simulink model "Opera_Delt_Angulos"  (R2014a)
settings: Solver=ode45  StartTime=0.0  StopTime=1  RelTol=1e-3
PreLoadFcn:
  | Fs=0.001;
  | Fc=0.0005;
InitFcn:
  | Fs=0.001;
  | Fc=0.0005;
undefined symbols (not defined in the file or in its folder): X, Y, Z
libraries: sm_lib x238, Fricciones x12, nesl_utility x10, powerlib x1
(part 1 of 5)
Description:
  | Modelo de un robot tipo Delta, con:
  | -Fricción en las articulaciones
  | -Con interpolador de orden 5 en el espacio operacional.
  | -Cinematica inversa
  | -Sigue una trayectoria dada de pick and place, y devuelve los torques.
settings Model: Creator=Sebastian Serna Palleja  LastModifiedBy=Sebastian
settings Model: ModifiedComment=|
  | Sebastian -- Mon Apr 11 18:42:01 2016 -- Version 1.108
  | Actualizacion pesos
settings Model: ModifiedHistory=|
  | Sebastian -- Mon Apr 11 18:42:01 2016 -- Version 1.108
  | Actualizacion pesos
  | 
  | Modelo con funcion de pick and place,
  | organizado, con interpolador en el espacio operacional de orden 5.
settings SolverCC: ConsecutiveZCsStepRelTol=10*100*eps  ZeroCrossControl=EnableAll  AutoInsertRateTranBlk=on

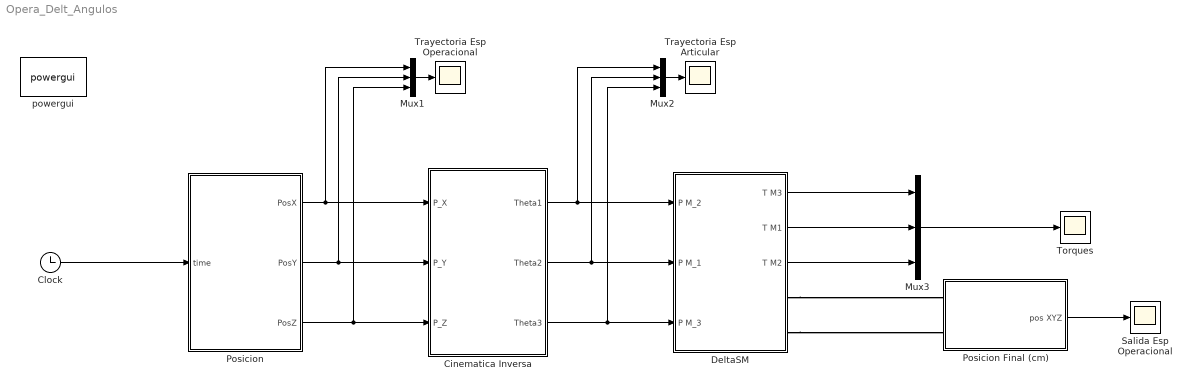
== system Opera_Delt_Angulos ==
  Cinematica Inversa : Subsystem
  Clock : Clock
  DeltaSM : Subsystem
  Mux1 : Mux  Inputs=3
  Mux2 : Mux  Inputs=3
  Mux3 : Mux  Inputs=3
  "Posicion " : MATLAB Function  TreatAsAtomicUnit=on
  Posicion Final (cm) : Subsystem
  Salida Esp Operacional : Scope
      settings: SaveName=ScopeData5
  Torques : Scope
      settings: YMin=-0.25  YMax=0.225  SaveName=Torque
  Trayectoria Esp Articular : Scope
      settings: SaveName=ScopeData4
  Trayectoria Esp Operacional : Scope
      settings: SaveName=ScopeData3
  powergui : powerlib/powergui  Priority=1  SimulationMode=Continuous  SolverType=Tustin  SampleTime=50e-6  frequency=60  SPID=off  DisableSnubberDevices=off  DisableRonSwitches=off  DisableVfSwitches=off  SwTol=0  Interpol=off  DisplayEquations=off  Ts=0  methode=off  frequencyindice=60  Pbase=100e6  ErrMax=1e-4  Iterations=50  UnitsV=kV  UnitsW=MW  FunctionMessages=off  echomessages=off  HookPort=off  EnableUseOfTLC=off  x0status=blocks  RestoreLinks=warning  ResistiveCurrentMeasurement=off  Frange=[0:2:500]  Ylog=off  Xlog=on  ShowGrid=off  save=off  variable=ZData  structure=0  ZoomFFT=off  StartTime=0.0  cycles=1  DisplayStyle=1  fundamental=60  FreqAxis=off  MaxFrequency=1000  frequencyindicesteady=1  RmsSteady=1  display=off
  wires:
  Posicion Final (cm)/1(pos XYZ) -> Salida Esp Operacional/1
  Clock/1 -> "Posicion "/1(time)
  Mux1/1 -> Trayectoria Esp Operacional/1
  Mux3/1 -> Torques/1
  DeltaSM/2(T M1) -> Mux3/2
  "Posicion "/3(PosZ) -> Mux1/3, Cinematica Inversa/3(P_Z)
  "Posicion "/2(PosY) -> Mux1/2, Cinematica Inversa/2(P_Y)
  "Posicion "/1(PosX) -> Cinematica Inversa/1(P_X), Mux1/1
  Mux2/1 -> Trayectoria Esp Articular/1
  Cinematica Inversa/3(Theta3) -> Mux2/3, DeltaSM/3(P M_3)
  Cinematica Inversa/2(Theta2) -> Mux2/2, DeltaSM/2(P M_1)
  Cinematica Inversa/1(Theta1) -> Mux2/1, DeltaSM/1(P M_2)
  DeltaSM/3(T M2) -> Mux3/3
  DeltaSM/1(T M3) -> Mux3/1
  connections:
  DeltaSM/RConn2 -- Posicion Final (cm)/LConn2
  DeltaSM/RConn1 -- Posicion Final (cm)/LConn1

== system Opera_Delt_Angulos/Cinematica Inversa ==
  P_X : Inport
  P_Y : Inport  Port=2
  P_Z : Inport  Port=3
  Cinematica Inversa : MATLAB Function  TreatAsAtomicUnit=on
  G_1 : Gain
  G_2 : Gain
  G_3 : Gain  Gain=-1
  Retardo1 : TransportDelay  DelayTime=0.01
  Retardo2 : TransportDelay  DelayTime=0.01
  Retardo3 : TransportDelay  DelayTime=0.01
  Theta1 : Outport
  Theta2 : Outport  Port=2
  Theta3 : Outport  Port=3
  wires:
  P_X/1 -> Cinematica Inversa/1(Px)
  P_Y/1 -> Cinematica Inversa/2(Py)
  Cinematica Inversa/3(ThetaM3) -> G_3/1, Retardo1/1
  Cinematica Inversa/1(ThetaM1) -> G_1/1, Retardo3/1
  Retardo2/1 -> Cinematica Inversa/5(AntThetaM2)
  Retardo3/1 -> Cinematica Inversa/4(AntThetaM1)
  Retardo1/1 -> Cinematica Inversa/6(AntThetaM3)
  Cinematica Inversa/2(ThetaM2) -> G_2/1, Retardo2/1
  G_1/1 -> Theta1/1
  G_2/1 -> Theta2/1
  G_3/1 -> Theta3/1
  P_Z/1 -> Cinematica Inversa/3(Pz)

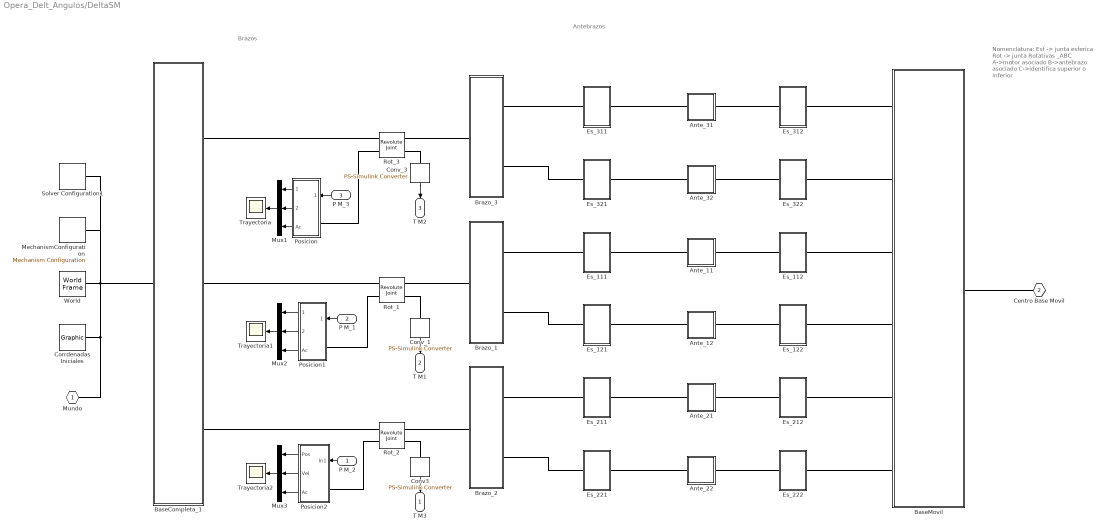
== system Opera_Delt_Angulos/DeltaSM ==
  note: Nomenclatura:
      | Esf  -> junta esferica
      | Rot -> junta Rotativas
      |
      | _ABC
      | A->motor asociado
      | B->antebrazo asociado
      | C->identifica superior o inferior
  note: Brazos
  note: Antebrazos
  P M_2 : Inport
  P M_1 : Inport  Port=2
  P M_3 : Inport  Port=3
  Ante_11 : Subsystem
  Ante_12 : Subsystem
  Ante_21 : Subsystem
  Ante_22 : Subsystem
  Ante_31 : Subsystem
  Ante_32 : Subsystem
  BaseCompleta_1 : Subsystem
  BaseMovil : Subsystem
  Brazo_1 : Subsystem
  Brazo_2 : Subsystem
  Brazo_3 : Subsystem
  Conv3 : nesl_utility/PS-Simulink Converter  PhysicalDomain=network_engine_domain  SubClassName=ps_output  LeftPortType=input  RightPortType=output  PseudoPeriodic=off  Frequencies=[]  Unit=N*m  AffineConversion=off
  Conv_1 : nesl_utility/PS-Simulink Converter  PhysicalDomain=network_engine_domain  SubClassName=ps_output  LeftPortType=input  RightPortType=output  PseudoPeriodic=off  Frequencies=[]  Unit=N*m  AffineConversion=off
  Conv_3 : nesl_utility/PS-Simulink Converter  PhysicalDomain=network_engine_domain  SubClassName=ps_output  LeftPortType=input  RightPortType=output  PseudoPeriodic=off  Frequencies=[]  Unit=N*m  AffineConversion=off
  "Corrdenadas Iniciales " : sm_lib/Body Elements/Graphic  GraphicType=Marker  MarkerShape=Frame  MarkerSize=25  MarkerSizeUnits=m  GraphicVisPropType=SimpleVisualProperties  GraphicDiffuseColor=[0.0 0.0 0.0]  GraphicSpecularColor=[0.2 0.2 0.2]  GraphicAmbientColor=[0.5 0.5 0.5]  GraphicEmissiveColor=[0.0 0.0 0.0 1.0]  GraphicShininess=24.0  GraphicOpacity=1.0  BlockFunction=simmechanics.library.body_elements.graphic
  Es_111 : Subsystem
  Es_112 : Subsystem
  Es_121 : Subsystem
  Es_122 : Subsystem
  Es_211 : Subsystem
  Es_212 : Subsystem
  Es_221 : Subsystem
  Es_222 : Subsystem
  Es_311 : Subsystem
  Es_312 : Subsystem
  Es_321 : Subsystem
  Es_322 : Subsystem
  MechanismConfiguration : sm_lib/Utilities/Mechanism Configuration  UniformGravity=Constant  GravityVector=[0 0 -9.81]  GravityUnits=m/s^2  LinearizationDelta=0.001  BlockFunction=simmechanics.library.utilities.mechanism_configuration
  Mux1 : Mux  Inputs=3
  Mux2 : Mux  Inputs=3
  Mux3 : Mux  Inputs=3
  Posicion : Subsystem
  Posicion1 : Subsystem
  Posicion2 : Subsystem
  Rot_1 : sm_lib/Joints/Revolute Joint  SenseConstraintForce=off  SenseConstraintForceX=off  SenseConstraintForceY=off  SenseConstraintForceZ=off  SenseConstraintTorque=off  SenseConstraintTorqueX=off  SenseConstraintTorqueY=off  SenseConstraintTorqueZ=off  SenseTotalForce=off  SenseTotalForceX=off  SenseTotalForceY=off  SenseTotalForceZ=off  SenseTotalTorque=off  SenseTotalTorqueX=off  SenseTotalTorqueY=off  SenseTotalTorqueZ=off  CompositeWrenchDir=FollowerOnBase  CompositeWrenchFrame=BaseFrame  EquilibriumPosition=0  EquilibriumPositionUnits=rad  SpringStiffness=0  SpringStiffnessUnits=m*N/rad  DampingCoefficient=0  DampingCoefficientUnits=m*s*N/rad  TorqueActuationMode=ComputedTorque  MotionActuationMode=InputMotion  SensePosition=off  SenseVelocity=off  SenseAcceleration=off  SenseTorqueForce=on  PositionTargetValue=-154.29618803259041  PositionTargetValueUnits=deg  PositionTargetSpecify=off  PositionTargetPriority=Low  VelocityTargetValue=0  VelocityTargetValueUnits=deg/s  VelocityTargetSpecify=off  VelocityTargetPriority=High  BlockFunction=simmechanics.library.joints.revolute_joint
  Rot_2 : sm_lib/Joints/Revolute Joint  SenseConstraintForce=off  SenseConstraintForceX=off  SenseConstraintForceY=off  SenseConstraintForceZ=off  SenseConstraintTorque=off  SenseConstraintTorqueX=off  SenseConstraintTorqueY=off  SenseConstraintTorqueZ=off  SenseTotalForce=off  SenseTotalForceX=off  SenseTotalForceY=off  SenseTotalForceZ=off  SenseTotalTorque=off  SenseTotalTorqueX=off  SenseTotalTorqueY=off  SenseTotalTorqueZ=off  CompositeWrenchDir=FollowerOnBase  CompositeWrenchFrame=BaseFrame  EquilibriumPosition=0  EquilibriumPositionUnits=rad  SpringStiffness=0  SpringStiffnessUnits=m*N/rad  DampingCoefficient=0  DampingCoefficientUnits=m*s*N/rad  TorqueActuationMode=ComputedTorque  MotionActuationMode=InputMotion  SensePosition=off  SenseVelocity=off  SenseAcceleration=off  SenseTorqueForce=on  PositionTargetValue=-72.758960975562829  PositionTargetValueUnits=deg  PositionTargetSpecify=off  PositionTargetPriority=Low  VelocityTargetValue=0  VelocityTargetValueUnits=deg/s  VelocityTargetSpecify=off  VelocityTargetPriority=High  BlockFunction=simmechanics.library.joints.revolute_joint
  Rot_3 : sm_lib/Joints/Revolute Joint  SenseConstraintForce=off  SenseConstraintForceX=off  SenseConstraintForceY=off  SenseConstraintForceZ=off  SenseConstraintTorque=off  SenseConstraintTorqueX=off  SenseConstraintTorqueY=off  SenseConstraintTorqueZ=off  SenseTotalForce=off  SenseTotalForceX=off  SenseTotalForceY=off  SenseTotalForceZ=off  SenseTotalTorque=off  SenseTotalTorqueX=off  SenseTotalTorqueY=off  SenseTotalTorqueZ=off  CompositeWrenchDir=FollowerOnBase  CompositeWrenchFrame=BaseFrame  EquilibriumPosition=0  EquilibriumPositionUnits=rad  SpringStiffness=0  SpringStiffnessUnits=m*N/rad  DampingCoefficient=0  DampingCoefficientUnits=m*s*N/rad  TorqueActuationMode=ComputedTorque  MotionActuationMode=InputMotion  SensePosition=off  SenseVelocity=off  SenseAcceleration=off  SenseTorqueForce=on  PositionTargetValue=0  PositionTargetValueUnits=deg  PositionTargetSpecify=off  PositionTargetPriority=Low  VelocityTargetValue=0  VelocityTargetValueUnits=deg/s  VelocityTargetSpecify=off  VelocityTargetPriority=High  BlockFunction=simmechanics.library.joints.revolute_joint
  Solver Configuration1 : nesl_utility/Solver Configuration  PhysicalDomain=network_engine_domain  SubClassName=solver  LeftPortType=input  RightPortType=generic  Accelerate=off  Tones=[]  Harmonics=[]  SimulateNoise=off  Profile=off  UseLocalSampling=off  EnableSwitchedLinearOptims=on  FrequencyDomain=off  UseCCode=off  RelTol=0.001  AbsTol=1e-06  MinStep=1e-09  ToWorkspace=off  DoDC=on  ResidualTolerance=1e-09  UseLocalSolver=on  LocalSolverChoice=NE_BACKWARD_EULER_ADVANCER  LocalSolverSampleTime=0.00005  DoFixedCost=on  MaxNonlinIter=50  MaxModeIter=2  LinearAlgebra=Full  DelaysMemoryBudget=2048  AutomaticFiltering=on  FilteringTimeConstant=0.001
  Trayectoria : Scope
  Trayectoria1 : Scope
      settings: YMin=-3  YMax=0
  Trayectoria2 : Scope
      settings: SaveName=ScopeData2
  World : sm_lib/Frames and Transforms/World Frame  BlockFunction=simmechanics.library.frames_transforms.world_frame
  Mundo : PMIOPort  Port=1  Side=Right
  Centro Base Movil : PMIOPort  Port=2  Side=Right
  T M3 : Outport
  T M1 : Outport  Port=2
  T M2 : Outport  Port=3
  wires:
  Conv_3/1 -> T M2/1
  P M_3/1 -> Posicion/1(In1)
  Mux1/1 -> Trayectoria/1
  Posicion/1(Pos) -> Mux1/1
  Posicion/2(Vel) -> Mux1/2
  Posicion/3(Ac) -> Mux1/3
  Conv_1/1 -> T M1/1
  P M_1/1 -> Posicion1/1(In1)
  Mux2/1 -> Trayectoria1/1
  Posicion1/3(Ac) -> Mux2/3
  Conv3/1 -> T M3/1
  P M_2/1 -> Posicion2/1(In1)
  Mux3/1 -> Trayectoria2/1
  Posicion2/1(Pos) -> Mux3/1
  Posicion2/2(Vel) -> Mux3/2
  Posicion2/3(Ac) -> Mux3/3
  Posicion1/2(Vel) -> Mux2/2
  Posicion1/1(Pos) -> Mux2/1
  connections:
  BaseCompleta_1/RConn2 -- Rot_1/LConn1
  Brazo_2/LConn1 -- Rot_2/RConn1
  BaseCompleta_1/RConn1 -- Rot_3/LConn1
  Brazo_3/LConn1 -- Rot_3/RConn1
  Brazo_1/LConn1 -- Rot_1/RConn1
  BaseCompleta_1/RConn3 -- Rot_2/LConn1
  "Corrdenadas Iniciales "/RConn1 -- Mundo/RConn1 -- BaseCompleta_1/LConn1 -- Solver Configuration1/RConn1 -- MechanismConfiguration/RConn1 -- World/RConn1
  Posicion/LConn1 -- Rot_3/LConn2
  Conv_3/LConn1 -- Rot_3/RConn2
  Posicion1/LConn1 -- Rot_1/LConn2
  Conv_1/LConn1 -- Rot_1/RConn2
  Posicion2/LConn1 -- Rot_2/LConn2
  Conv3/LConn1 -- Rot_2/RConn2
  BaseMovil/RConn1 -- Centro Base Movil/RConn1
  Ante_31/LConn1 -- Es_311/RConn1
  Ante_21/RConn1 -- Es_212/LConn1
  BaseMovil/LConn3 -- Es_112/RConn1
  BaseMovil/LConn2 -- Es_322/RConn1
  Brazo_1/RConn2 -- Es_121/LConn1
  Brazo_3/RConn2 -- Es_321/LConn1
  Ante_21/LConn1 -- Es_211/RConn1
  BaseMovil/LConn6 -- Es_222/RConn1
  Ante_22/LConn1 -- Es_221/RConn1
  Brazo_1/RConn1 -- Es_111/LConn1
  Ante_32/LConn1 -- Es_321/RConn1
  Ante_32/RConn1 -- Es_322/LConn1
  Brazo_2/RConn1 -- Es_211/LConn1
  Ante_22/RConn1 -- Es_222/LConn1
  BaseMovil/LConn1 -- Es_312/RConn1
  BaseMovil/LConn5 -- Es_212/RConn1
  Ante_12/RConn1 -- Es_122/LConn1
  Ante_31/RConn1 -- Es_312/LConn1
  Ante_11/LConn1 -- Es_111/RConn1
  BaseMovil/LConn4 -- Es_122/RConn1
  Brazo_2/RConn2 -- Es_221/LConn1
  Ante_12/LConn1 -- Es_121/RConn1
  Ante_11/RConn1 -- Es_112/LConn1
  Brazo_3/RConn1 -- Es_311/LConn1

== system Opera_Delt_Angulos/Posicion Final (cm) ==
  M1 : Scope
      settings: SaveName=ScopeData7
  M2 : Scope
      settings: SaveName=ScopeData8
  "M3 " : Scope
      settings: SaveName=ScopeData6
  Mux : Mux  Inputs=3
  Pos X Converter : nesl_utility/PS-Simulink Converter  PhysicalDomain=network_engine_domain  SubClassName=ps_output  LeftPortType=input  RightPortType=output  PseudoPeriodic=off  Frequencies=[]  Unit=mm  AffineConversion=off
  Pos Y Converter1 : nesl_utility/PS-Simulink Converter  PhysicalDomain=network_engine_domain  SubClassName=ps_output  LeftPortType=input  RightPortType=output  PseudoPeriodic=off  Frequencies=[]  Unit=mm  AffineConversion=off
  Pos Z Converter2 : nesl_utility/PS-Simulink Converter  PhysicalDomain=network_engine_domain  SubClassName=ps_output  LeftPortType=input  RightPortType=output  PseudoPeriodic=off  Frequencies=[]  Unit=mm  AffineConversion=off
  Transform Sensor : sm_lib/Frames and Transforms/Transform Sensor  MeasurementFrame=World  SenseAngle=off  SenseAxis=off  SenseAngle1=off  SenseAngle2=off  SenseAngle3=off  SenseQ=off  SenseR=off  SenseOmegaX=off  SenseOmegaY=off  SenseOmegaZ=off  SenseOmega1=off  SenseOmega2=off  SenseOmega3=off  SenseQDot=off  SenseRDot=off  SenseAlphaX=off  SenseAlphaY=off  SenseAlphaZ=off  SenseAlpha1=off  SenseAlpha2=off  SenseAlpha3=off  SenseQDDot=off  SenseRDDot=off  SenseX=on  SenseY=on  SenseZ=on  SenseRad=off  SenseAzim=off  SenseDist=off  SenseInc=off  SenseXDot=off  SenseYDot=off  SenseZDot=off  SenseRadDot=off  SenseAzimDot=off  SenseDistDot=off  SenseIncDot=off  SenseXDDot=off  SenseYDDot=off  SenseZDDot=off  SenseRadDDot=off  SenseAzimDDot=off  SenseDistDDot=off  SenseIncDDot=off  BlockFunction=simmechanics.library.frames_transforms.transform_sensor
  world : PMIOPort  Port=1  Side=Left
  Centro Base Movil : PMIOPort  Port=2  Side=Left
  pos XYZ : Outport
  wires:
  Pos Z Converter2/1 -> M2/1, Mux/3
  Mux/1 -> pos XYZ/1
  Pos Y Converter1/1 -> M1/1, Mux/2
  Pos X Converter/1 -> Mux/1, "M3 "/1
  connections:
  world/RConn1 -- Transform Sensor/LConn1
  Pos Z Converter2/LConn1 -- Transform Sensor/RConn4
  Transform Sensor/RConn2 -- Pos X Converter/LConn1
  Pos Y Converter1/LConn1 -- Transform Sensor/RConn3
  Centro Base Movil/RConn1 -- Transform Sensor/RConn1

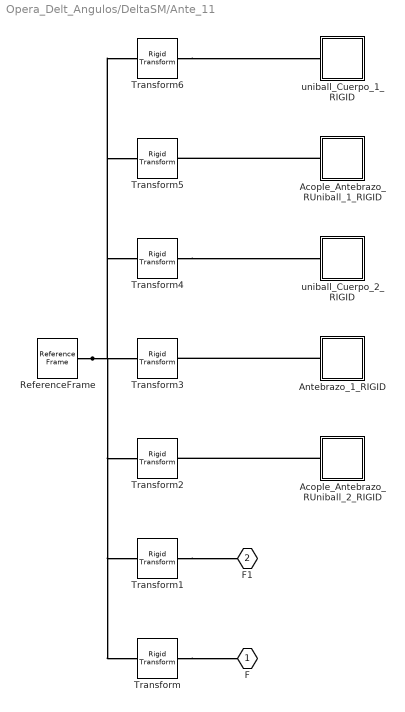
== system Opera_Delt_Angulos/DeltaSM/Ante_11 ==
  Acople_Antebrazo_RUniball_1_RIGID : Subsystem
  Acople_Antebrazo_RUniball_2_RIGID : Subsystem
  Antebrazo_1_RIGID : Subsystem
  ReferenceFrame : sm_lib/Frames and Transforms/Reference Frame  BlockFunction=simmechanics.library.frames_transforms.reference_frame
  Transform : sm_lib/Frames and Transforms/Rigid Transform  TranslationMethod=Cartesian  TranslationLengthUnit=mm  TranslationStandardAxis=+Z  TranslationStandardOffset=0  TranslationCartesianOffset=[-16.089268306127384 11.758961591624281 40.649351392904187]  TranslationROffset=0  TranslationROffsetUnits=m  TranslationZOffset=0  TranslationZOffsetUnits=m  TranslationThetaOffset=0  TranslationThetaOffsetUnits=deg  RotationMethod=ArbitraryAxis  RotationAngleUnits=rad  RotationStandardAxis=+Z  RotationAngle=0  RotationArbitraryAxis=[0 0 0]  FollAlignAxisA=+X  BaseAlignAxisA=+Y  FollAlignAxisB=+Y  BaseAlignAxisB=+Z  BlockFunction=simmechanics.library.frames_transforms.rigid_transform
  Transform1 : sm_lib/Frames and Transforms/Rigid Transform  TranslationMethod=Cartesian  TranslationLengthUnit=mm  TranslationStandardAxis=+Z  TranslationStandardOffset=0  TranslationCartesianOffset=[-16.089268306127369 -263.24103840837563 40.649351392904151]  TranslationROffset=0  TranslationROffsetUnits=m  TranslationZOffset=0  TranslationZOffsetUnits=m  TranslationThetaOffset=0  TranslationThetaOffsetUnits=deg  RotationMethod=ArbitraryAxis  RotationAngleUnits=rad  RotationStandardAxis=+Z  RotationAngle=0  RotationArbitraryAxis=[0 0 0]  FollAlignAxisA=+X  BaseAlignAxisA=+Y  FollAlignAxisB=+Y  BaseAlignAxisB=+Z  BlockFunction=simmechanics.library.frames_transforms.rigid_transform
  Transform2 : sm_lib/Frames and Transforms/Rigid Transform  TranslationMethod=Cartesian  TranslationLengthUnit=mm  TranslationStandardAxis=+Z  TranslationStandardOffset=0  TranslationCartesianOffset=[-16.089268306127376 -51.741038408375687 40.649351392904165]  TranslationROffset=0  TranslationROffsetUnits=m  TranslationZOffset=0  TranslationZOffsetUnits=m  TranslationThetaOffset=0  TranslationThetaOffsetUnits=deg  RotationMethod=ArbitraryAxis  RotationAngleUnits=rad  RotationStandardAxis=+Z  RotationAngle=2.7352803968007873  RotationArbitraryAxis=[-0.2059979679735047 0.69194105138761164 0.69194105138761175]  FollAlignAxisA=+X  BaseAlignAxisA=+Y  FollAlignAxisB=+Y  BaseAlignAxisB=+Z  BlockFunction=simmechanics.library.frames_transforms.rigid_transform
  Transform3 : sm_lib/Frames and Transforms/Rigid Transform  TranslationMethod=Cartesian  TranslationLengthUnit=mm  TranslationStandardAxis=+Z  TranslationStandardOffset=0  TranslationCartesianOffset=[-16.089268306127384 -227.74103840837574 40.64935139290418]  TranslationROffset=0  TranslationROffsetUnits=m  TranslationZOffset=0  TranslationZOffsetUnits=m  TranslationThetaOffset=0  TranslationThetaOffsetUnits=deg  RotationMethod=ArbitraryAxis  RotationAngleUnits=rad  RotationStandardAxis=+Z  RotationAngle=2.7352803968007873  RotationArbitraryAxis=[-0.2059979679735047 0.69194105138761164 0.69194105138761175]  FollAlignAxisA=+X  BaseAlignAxisA=+Y  FollAlignAxisB=+Y  BaseAlignAxisB=+Z  BlockFunction=simmechanics.library.frames_transforms.rigid_transform
  Transform4 : sm_lib/Frames and Transforms/Rigid Transform  TranslationMethod=Cartesian  TranslationLengthUnit=mm  TranslationStandardAxis=+Z  TranslationStandardOffset=0  TranslationCartesianOffset=[-16.089268306127369 -263.24103840837563 40.649351392904151]  TranslationROffset=0  TranslationROffsetUnits=m  TranslationZOffset=0  TranslationZOffsetUnits=m  TranslationThetaOffset=0  TranslationThetaOffsetUnits=deg  RotationMethod=ArbitraryAxis  RotationAngleUnits=rad  RotationStandardAxis=+Z  RotationAngle=3.1415926535897931  RotationArbitraryAxis=[-1.1188966420050406e-16 0 1]  FollAlignAxisA=+X  BaseAlignAxisA=+Y  FollAlignAxisB=+Y  BaseAlignAxisB=+Z  BlockFunction=simmechanics.library.frames_transforms.rigid_transform
  Transform5 : sm_lib/Frames and Transforms/Rigid Transform  TranslationMethod=Cartesian  TranslationLengthUnit=mm  TranslationStandardAxis=+Z  TranslationStandardOffset=0  TranslationCartesianOffset=[-16.089268306127391 -199.7410384083758 40.64935139290418]  TranslationROffset=0  TranslationROffsetUnits=m  TranslationZOffset=0  TranslationZOffsetUnits=m  TranslationThetaOffset=0  TranslationThetaOffsetUnits=deg  RotationMethod=ArbitraryAxis  RotationAngleUnits=rad  RotationStandardAxis=+Z  RotationAngle=2.7352803968007873  RotationArbitraryAxis=[0.2059979679735047 0.69194105138761164 -0.69194105138761175]  FollAlignAxisA=+X  BaseAlignAxisA=+Y  FollAlignAxisB=+Y  BaseAlignAxisB=+Z  BlockFunction=simmechanics.library.frames_transforms.rigid_transform
  Transform6 : sm_lib/Frames and Transforms/Rigid Transform  TranslationMethod=Cartesian  TranslationLengthUnit=mm  TranslationStandardAxis=+Z  TranslationStandardOffset=0  TranslationCartesianOffset=[-16.089268306127376 11.758961591624317 40.649351392904165]  TranslationROffset=0  TranslationROffsetUnits=m  TranslationZOffset=0  TranslationZOffsetUnits=m  TranslationThetaOffset=0  TranslationThetaOffsetUnits=deg  RotationMethod=None  RotationAngleUnits=deg  RotationStandardAxis=+Z  RotationAngle=0  RotationArbitraryAxis=[0 0 1]  FollAlignAxisA=+X  BaseAlignAxisA=+Y  FollAlignAxisB=+Y  BaseAlignAxisB=+Z  BlockFunction=simmechanics.library.frames_transforms.rigid_transform
  uniball_Cuerpo_1_RIGID : Subsystem
  uniball_Cuerpo_2_RIGID : Subsystem
  F : PMIOPort  Port=1  Side=Left
  F1 : PMIOPort  Port=2  Side=Right
  connections:
  ReferenceFrame/RConn1 -- Transform/LConn1 -- Transform1/LConn1 -- Transform2/LConn1 -- Transform3/LConn1 -- Transform4/LConn1 -- Transform5/LConn1 -- Transform6/LConn1
  Transform/RConn1 -- F/RConn1
  Transform1/RConn1 -- F1/RConn1
  Acople_Antebrazo_RUniball_2_RIGID/LConn1 -- Transform2/RConn1
  Antebrazo_1_RIGID/LConn1 -- Transform3/RConn1
  Transform4/RConn1 -- uniball_Cuerpo_2_RIGID/LConn1
  Acople_Antebrazo_RUniball_1_RIGID/LConn1 -- Transform5/RConn1
  Transform6/RConn1 -- uniball_Cuerpo_1_RIGID/LConn1

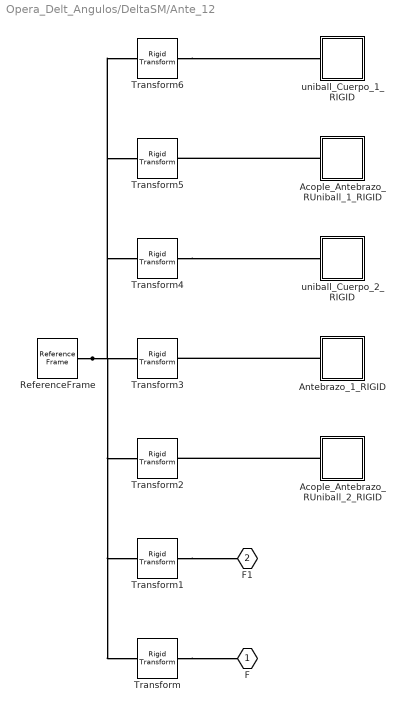
== system Opera_Delt_Angulos/DeltaSM/Ante_12 ==
  Acople_Antebrazo_RUniball_1_RIGID : Subsystem
  Acople_Antebrazo_RUniball_2_RIGID : Subsystem
  Antebrazo_1_RIGID : Subsystem
  ReferenceFrame : sm_lib/Frames and Transforms/Reference Frame  BlockFunction=simmechanics.library.frames_transforms.reference_frame
  Transform : sm_lib/Frames and Transforms/Rigid Transform  TranslationMethod=Cartesian  TranslationLengthUnit=mm  TranslationStandardAxis=+Z  TranslationStandardOffset=0  TranslationCartesianOffset=[-16.089268306127394 11.758961591624296 40.64935139290418]  TranslationROffset=0  TranslationROffsetUnits=m  TranslationZOffset=0  TranslationZOffsetUnits=m  TranslationThetaOffset=0  TranslationThetaOffsetUnits=deg  RotationMethod=ArbitraryAxis  RotationAngleUnits=rad  RotationStandardAxis=+Z  RotationAngle=0  RotationArbitraryAxis=[0 0 0]  FollAlignAxisA=+X  BaseAlignAxisA=+Y  FollAlignAxisB=+Y  BaseAlignAxisB=+Z  BlockFunction=simmechanics.library.frames_transforms.rigid_transform
  Transform1 : sm_lib/Frames and Transforms/Rigid Transform  TranslationMethod=Cartesian  TranslationLengthUnit=mm  TranslationStandardAxis=+Z  TranslationStandardOffset=0  TranslationCartesianOffset=[-16.089268306127391 -263.24103840837574 40.649351392904165]  TranslationROffset=0  TranslationROffsetUnits=m  TranslationZOffset=0  TranslationZOffsetUnits=m  TranslationThetaOffset=0  TranslationThetaOffsetUnits=deg  RotationMethod=ArbitraryAxis  RotationAngleUnits=rad  RotationStandardAxis=+Z  RotationAngle=0  RotationArbitraryAxis=[0 0 0]  FollAlignAxisA=+X  BaseAlignAxisA=+Y  FollAlignAxisB=+Y  BaseAlignAxisB=+Z  BlockFunction=simmechanics.library.frames_transforms.rigid_transform
  Transform2 : sm_lib/Frames and Transforms/Rigid Transform  TranslationMethod=Cartesian  TranslationLengthUnit=mm  TranslationStandardAxis=+Z  TranslationStandardOffset=0  TranslationCartesianOffset=[-16.089268306127362 -51.741038408375672 40.64935139290418]  TranslationROffset=0  TranslationROffsetUnits=m  TranslationZOffset=0  TranslationZOffsetUnits=m  TranslationThetaOffset=0  TranslationThetaOffsetUnits=deg  RotationMethod=ArbitraryAxis  RotationAngleUnits=rad  RotationStandardAxis=+Z  RotationAngle=2.7352803968007873  RotationArbitraryAxis=[-0.20599796797350473 0.69194105138761164 0.69194105138761175]  FollAlignAxisA=+X  BaseAlignAxisA=+Y  FollAlignAxisB=+Y  BaseAlignAxisB=+Z  BlockFunction=simmechanics.library.frames_transforms.rigid_transform
  Transform3 : sm_lib/Frames and Transforms/Rigid Transform  TranslationMethod=Cartesian  TranslationLengthUnit=mm  TranslationStandardAxis=+Z  TranslationStandardOffset=0  TranslationCartesianOffset=[-16.089268306127376 -227.74103840837577 40.64935139290418]  TranslationROffset=0  TranslationROffsetUnits=m  TranslationZOffset=0  TranslationZOffsetUnits=m  TranslationThetaOffset=0  TranslationThetaOffsetUnits=deg  RotationMethod=ArbitraryAxis  RotationAngleUnits=rad  RotationStandardAxis=+Z  RotationAngle=2.7352803968007873  RotationArbitraryAxis=[-0.20599796797350473 0.69194105138761164 0.69194105138761175]  FollAlignAxisA=+X  BaseAlignAxisA=+Y  FollAlignAxisB=+Y  BaseAlignAxisB=+Z  BlockFunction=simmechanics.library.frames_transforms.rigid_transform
  Transform4 : sm_lib/Frames and Transforms/Rigid Transform  TranslationMethod=Cartesian  TranslationLengthUnit=mm  TranslationStandardAxis=+Z  TranslationStandardOffset=0  TranslationCartesianOffset=[-16.089268306127391 -263.24103840837574 40.649351392904165]  TranslationROffset=0  TranslationROffsetUnits=m  TranslationZOffset=0  TranslationZOffsetUnits=m  TranslationThetaOffset=0  TranslationThetaOffsetUnits=deg  RotationMethod=ArbitraryAxis  RotationAngleUnits=rad  RotationStandardAxis=+Z  RotationAngle=3.1415926535897931  RotationArbitraryAxis=[-1.1188966420050406e-16 0 1]  FollAlignAxisA=+X  BaseAlignAxisA=+Y  FollAlignAxisB=+Y  BaseAlignAxisB=+Z  BlockFunction=simmechanics.library.frames_transforms.rigid_transform
  Transform5 : sm_lib/Frames and Transforms/Rigid Transform  TranslationMethod=Cartesian  TranslationLengthUnit=mm  TranslationStandardAxis=+Z  TranslationStandardOffset=0  TranslationCartesianOffset=[-16.089268306127376 -199.74103840837577 40.649351392904165]  TranslationROffset=0  TranslationROffsetUnits=m  TranslationZOffset=0  TranslationZOffsetUnits=m  TranslationThetaOffset=0  TranslationThetaOffsetUnits=deg  RotationMethod=ArbitraryAxis  RotationAngleUnits=rad  RotationStandardAxis=+Z  RotationAngle=2.7352803968007873  RotationArbitraryAxis=[0.20599796797350473 0.69194105138761164 -0.69194105138761175]  FollAlignAxisA=+X  BaseAlignAxisA=+Y  FollAlignAxisB=+Y  BaseAlignAxisB=+Z  BlockFunction=simmechanics.library.frames_transforms.rigid_transform
  Transform6 : sm_lib/Frames and Transforms/Rigid Transform  TranslationMethod=Cartesian  TranslationLengthUnit=mm  TranslationStandardAxis=+Z  TranslationStandardOffset=0  TranslationCartesianOffset=[-16.089268306127376 11.758961591624317 40.649351392904165]  TranslationROffset=0  TranslationROffsetUnits=m  TranslationZOffset=0  TranslationZOffsetUnits=m  TranslationThetaOffset=0  TranslationThetaOffsetUnits=deg  RotationMethod=None  RotationAngleUnits=deg  RotationStandardAxis=+Z  RotationAngle=0  RotationArbitraryAxis=[0 0 1]  FollAlignAxisA=+X  BaseAlignAxisA=+Y  FollAlignAxisB=+Y  BaseAlignAxisB=+Z  BlockFunction=simmechanics.library.frames_transforms.rigid_transform
  uniball_Cuerpo_1_RIGID : Subsystem
  uniball_Cuerpo_2_RIGID : Subsystem
  F : PMIOPort  Port=1  Side=Left
  F1 : PMIOPort  Port=2  Side=Right
  connections:
  ReferenceFrame/RConn1 -- Transform/LConn1 -- Transform1/LConn1 -- Transform2/LConn1 -- Transform3/LConn1 -- Transform4/LConn1 -- Transform5/LConn1 -- Transform6/LConn1
  Transform/RConn1 -- F/RConn1
  Transform1/RConn1 -- F1/RConn1
  Acople_Antebrazo_RUniball_2_RIGID/LConn1 -- Transform2/RConn1
  Antebrazo_1_RIGID/LConn1 -- Transform3/RConn1
  Transform4/RConn1 -- uniball_Cuerpo_2_RIGID/LConn1
  Acople_Antebrazo_RUniball_1_RIGID/LConn1 -- Transform5/RConn1
  Transform6/RConn1 -- uniball_Cuerpo_1_RIGID/LConn1

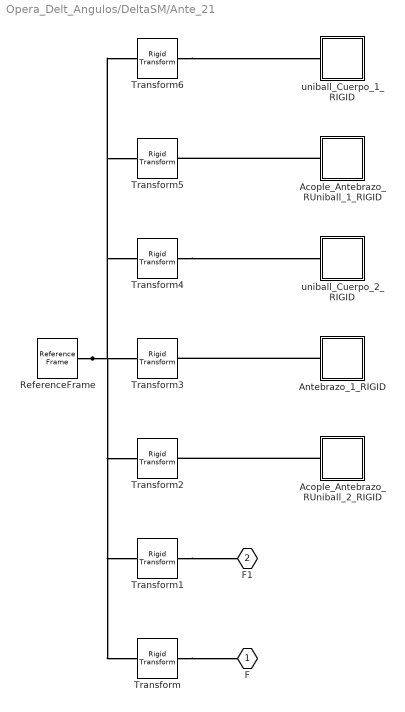
== system Opera_Delt_Angulos/DeltaSM/Ante_21 ==
  Acople_Antebrazo_RUniball_1_RIGID : Subsystem
  Acople_Antebrazo_RUniball_2_RIGID : Subsystem
  Antebrazo_1_RIGID : Subsystem
  ReferenceFrame : sm_lib/Frames and Transforms/Reference Frame  BlockFunction=simmechanics.library.frames_transforms.reference_frame
  Transform : sm_lib/Frames and Transforms/Rigid Transform  TranslationMethod=Cartesian  TranslationLengthUnit=mm  TranslationStandardAxis=+Z  TranslationStandardOffset=0  TranslationCartesianOffset=[-16.089268306127366 11.758961591624313 40.649351392904201]  TranslationROffset=0  TranslationROffsetUnits=m  TranslationZOffset=0  TranslationZOffsetUnits=m  TranslationThetaOffset=0  TranslationThetaOffsetUnits=deg  RotationMethod=ArbitraryAxis  RotationAngleUnits=rad  RotationStandardAxis=+Z  RotationAngle=0  RotationArbitraryAxis=[0 0 0]  FollAlignAxisA=+X  BaseAlignAxisA=+Y  FollAlignAxisB=+Y  BaseAlignAxisB=+Z  BlockFunction=simmechanics.library.frames_transforms.rigid_transform
  Transform1 : sm_lib/Frames and Transforms/Rigid Transform  TranslationMethod=Cartesian  TranslationLengthUnit=mm  TranslationStandardAxis=+Z  TranslationStandardOffset=0  TranslationCartesianOffset=[-16.089268306127362 -263.24103840837574 40.649351392904165]  TranslationROffset=0  TranslationROffsetUnits=m  TranslationZOffset=0  TranslationZOffsetUnits=m  TranslationThetaOffset=0  TranslationThetaOffsetUnits=deg  RotationMethod=ArbitraryAxis  RotationAngleUnits=rad  RotationStandardAxis=+Z  RotationAngle=0  RotationArbitraryAxis=[0 0 0]  FollAlignAxisA=+X  BaseAlignAxisA=+Y  FollAlignAxisB=+Y  BaseAlignAxisB=+Z  BlockFunction=simmechanics.library.frames_transforms.rigid_transform
  Transform2 : sm_lib/Frames and Transforms/Rigid Transform  TranslationMethod=Cartesian  TranslationLengthUnit=mm  TranslationStandardAxis=+Z  TranslationStandardOffset=0  TranslationCartesianOffset=[-16.089268306127376 -51.741038408375708 40.649351392904165]  TranslationROffset=0  TranslationROffsetUnits=m  TranslationZOffset=0  TranslationZOffsetUnits=m  TranslationThetaOffset=0  TranslationThetaOffsetUnits=deg  RotationMethod=ArbitraryAxis  RotationAngleUnits=rad  RotationStandardAxis=+Z  RotationAngle=2.7352803968007873  RotationArbitraryAxis=[-0.20599796797350473 0.69194105138761164 0.69194105138761175]  FollAlignAxisA=+X  BaseAlignAxisA=+Y  FollAlignAxisB=+Y  BaseAlignAxisB=+Z  BlockFunction=simmechanics.library.frames_transforms.rigid_transform
  Transform3 : sm_lib/Frames and Transforms/Rigid Transform  TranslationMethod=Cartesian  TranslationLengthUnit=mm  TranslationStandardAxis=+Z  TranslationStandardOffset=0  TranslationCartesianOffset=[-16.089268306127362 -227.74103840837572 40.649351392904173]  TranslationROffset=0  TranslationROffsetUnits=m  TranslationZOffset=0  TranslationZOffsetUnits=m  TranslationThetaOffset=0  TranslationThetaOffsetUnits=deg  RotationMethod=ArbitraryAxis  RotationAngleUnits=rad  RotationStandardAxis=+Z  RotationAngle=2.7352803968007873  RotationArbitraryAxis=[-0.20599796797350473 0.69194105138761164 0.69194105138761175]  FollAlignAxisA=+X  BaseAlignAxisA=+Y  FollAlignAxisB=+Y  BaseAlignAxisB=+Z  BlockFunction=simmechanics.library.frames_transforms.rigid_transform
  Transform4 : sm_lib/Frames and Transforms/Rigid Transform  TranslationMethod=Cartesian  TranslationLengthUnit=mm  TranslationStandardAxis=+Z  TranslationStandardOffset=0  TranslationCartesianOffset=[-16.089268306127362 -263.24103840837574 40.649351392904165]  TranslationROffset=0  TranslationROffsetUnits=m  TranslationZOffset=0  TranslationZOffsetUnits=m  TranslationThetaOffset=0  TranslationThetaOffsetUnits=deg  RotationMethod=ArbitraryAxis  RotationAngleUnits=rad  RotationStandardAxis=+Z  RotationAngle=3.1415926535897931  RotationArbitraryAxis=[-1.110223024625157e-16 0 1]  FollAlignAxisA=+X  BaseAlignAxisA=+Y  FollAlignAxisB=+Y  BaseAlignAxisB=+Z  BlockFunction=simmechanics.library.frames_transforms.rigid_transform
  Transform5 : sm_lib/Frames and Transforms/Rigid Transform  TranslationMethod=Cartesian  TranslationLengthUnit=mm  TranslationStandardAxis=+Z  TranslationStandardOffset=0  TranslationCartesianOffset=[-16.089268306127362 -199.74103840837569 40.649351392904165]  TranslationROffset=0  TranslationROffsetUnits=m  TranslationZOffset=0  TranslationZOffsetUnits=m  TranslationThetaOffset=0  TranslationThetaOffsetUnits=deg  RotationMethod=ArbitraryAxis  RotationAngleUnits=rad  RotationStandardAxis=+Z  RotationAngle=2.7352803968007873  RotationArbitraryAxis=[0.20599796797350473 0.69194105138761164 -0.69194105138761175]  FollAlignAxisA=+X  BaseAlignAxisA=+Y  FollAlignAxisB=+Y  BaseAlignAxisB=+Z  BlockFunction=simmechanics.library.frames_transforms.rigid_transform
  Transform6 : sm_lib/Frames and Transforms/Rigid Transform  TranslationMethod=Cartesian  TranslationLengthUnit=mm  TranslationStandardAxis=+Z  TranslationStandardOffset=0  TranslationCartesianOffset=[-16.089268306127391 11.758961591624317 40.649351392904165]  TranslationROffset=0  TranslationROffsetUnits=m  TranslationZOffset=0  TranslationZOffsetUnits=m  TranslationThetaOffset=0  TranslationThetaOffsetUnits=deg  RotationMethod=None  RotationAngleUnits=deg  RotationStandardAxis=+Z  RotationAngle=0  RotationArbitraryAxis=[0 0 1]  FollAlignAxisA=+X  BaseAlignAxisA=+Y  FollAlignAxisB=+Y  BaseAlignAxisB=+Z  BlockFunction=simmechanics.library.frames_transforms.rigid_transform
  uniball_Cuerpo_1_RIGID : Subsystem
  uniball_Cuerpo_2_RIGID : Subsystem
  F : PMIOPort  Port=1  Side=Left
  F1 : PMIOPort  Port=2  Side=Right
  connections:
  ReferenceFrame/RConn1 -- Transform/LConn1 -- Transform1/LConn1 -- Transform2/LConn1 -- Transform3/LConn1 -- Transform4/LConn1 -- Transform5/LConn1 -- Transform6/LConn1
  Transform/RConn1 -- F/RConn1
  Transform1/RConn1 -- F1/RConn1
  Acople_Antebrazo_RUniball_2_RIGID/LConn1 -- Transform2/RConn1
  Antebrazo_1_RIGID/LConn1 -- Transform3/RConn1
  Transform4/RConn1 -- uniball_Cuerpo_2_RIGID/LConn1
  Acople_Antebrazo_RUniball_1_RIGID/LConn1 -- Transform5/RConn1
  Transform6/RConn1 -- uniball_Cuerpo_1_RIGID/LConn1

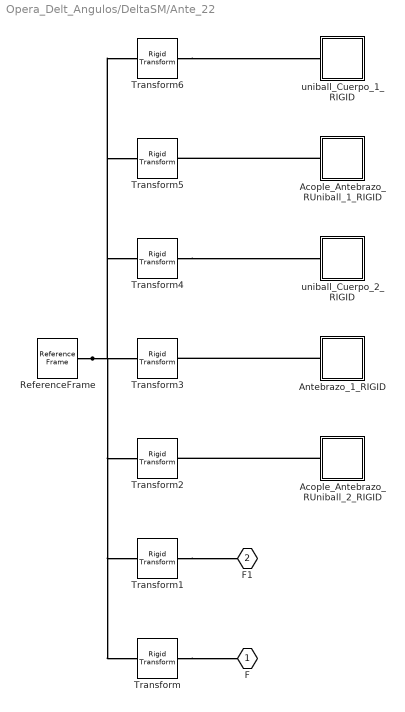
== system Opera_Delt_Angulos/DeltaSM/Ante_22 ==
  Acople_Antebrazo_RUniball_1_RIGID : Subsystem
  Acople_Antebrazo_RUniball_2_RIGID : Subsystem
  Antebrazo_1_RIGID : Subsystem
  ReferenceFrame : sm_lib/Frames and Transforms/Reference Frame  BlockFunction=simmechanics.library.frames_transforms.reference_frame
  Transform : sm_lib/Frames and Transforms/Rigid Transform  TranslationMethod=Cartesian  TranslationLengthUnit=mm  TranslationStandardAxis=+Z  TranslationStandardOffset=0  TranslationCartesianOffset=[-16.089268306127348 11.758961591624182 40.649351392904187]  TranslationROffset=0  TranslationROffsetUnits=m  TranslationZOffset=0  TranslationZOffsetUnits=m  TranslationThetaOffset=0  TranslationThetaOffsetUnits=deg  RotationMethod=ArbitraryAxis  RotationAngleUnits=rad  RotationStandardAxis=+Z  RotationAngle=0  RotationArbitraryAxis=[0 0 0]  FollAlignAxisA=+X  BaseAlignAxisA=+Y  FollAlignAxisB=+Y  BaseAlignAxisB=+Z  BlockFunction=simmechanics.library.frames_transforms.rigid_transform
  Transform1 : sm_lib/Frames and Transforms/Rigid Transform  TranslationMethod=Cartesian  TranslationLengthUnit=mm  TranslationStandardAxis=+Z  TranslationStandardOffset=0  TranslationCartesianOffset=[-16.089268306127391 -263.24103840837586 40.64935139290418]  TranslationROffset=0  TranslationROffsetUnits=m  TranslationZOffset=0  TranslationZOffsetUnits=m  TranslationThetaOffset=0  TranslationThetaOffsetUnits=deg  RotationMethod=ArbitraryAxis  RotationAngleUnits=rad  RotationStandardAxis=+Z  RotationAngle=0  RotationArbitraryAxis=[0 0 0]  FollAlignAxisA=+X  BaseAlignAxisA=+Y  FollAlignAxisB=+Y  BaseAlignAxisB=+Z  BlockFunction=simmechanics.library.frames_transforms.rigid_transform
  Transform2 : sm_lib/Frames and Transforms/Rigid Transform  TranslationMethod=Cartesian  TranslationLengthUnit=mm  TranslationStandardAxis=+Z  TranslationStandardOffset=0  TranslationCartesianOffset=[-16.089268306127391 -51.741038408375701 40.64935139290418]  TranslationROffset=0  TranslationROffsetUnits=m  TranslationZOffset=0  TranslationZOffsetUnits=m  TranslationThetaOffset=0  TranslationThetaOffsetUnits=deg  RotationMethod=ArbitraryAxis  RotationAngleUnits=rad  RotationStandardAxis=+Z  RotationAngle=2.7352803968007873  RotationArbitraryAxis=[-0.20599796797350467 0.69194105138761164 0.69194105138761164]  FollAlignAxisA=+X  BaseAlignAxisA=+Y  FollAlignAxisB=+Y  BaseAlignAxisB=+Z  BlockFunction=simmechanics.library.frames_transforms.rigid_transform
  Transform3 : sm_lib/Frames and Transforms/Rigid Transform  TranslationMethod=Cartesian  TranslationLengthUnit=mm  TranslationStandardAxis=+Z  TranslationStandardOffset=0  TranslationCartesianOffset=[-16.089268306127405 -227.74103840837577 40.64935139290418]  TranslationROffset=0  TranslationROffsetUnits=m  TranslationZOffset=0  TranslationZOffsetUnits=m  TranslationThetaOffset=0  TranslationThetaOffsetUnits=deg  RotationMethod=ArbitraryAxis  RotationAngleUnits=rad  RotationStandardAxis=+Z  RotationAngle=2.7352803968007873  RotationArbitraryAxis=[-0.20599796797350467 0.69194105138761164 0.69194105138761164]  FollAlignAxisA=+X  BaseAlignAxisA=+Y  FollAlignAxisB=+Y  BaseAlignAxisB=+Z  BlockFunction=simmechanics.library.frames_transforms.rigid_transform
  Transform4 : sm_lib/Frames and Transforms/Rigid Transform  TranslationMethod=Cartesian  TranslationLengthUnit=mm  TranslationStandardAxis=+Z  TranslationStandardOffset=0  TranslationCartesianOffset=[-16.089268306127391 -263.24103840837586 40.64935139290418]  TranslationROffset=0  TranslationROffsetUnits=m  TranslationZOffset=0  TranslationZOffsetUnits=m  TranslationThetaOffset=0  TranslationThetaOffsetUnits=deg  RotationMethod=ArbitraryAxis  RotationAngleUnits=rad  RotationStandardAxis=+Z  RotationAngle=3.1415926535897931  RotationArbitraryAxis=[-9.0856142054285235e-17 0 1]  FollAlignAxisA=+X  BaseAlignAxisA=+Y  FollAlignAxisB=+Y  BaseAlignAxisB=+Z  BlockFunction=simmechanics.library.frames_transforms.rigid_transform
  Transform5 : sm_lib/Frames and Transforms/Rigid Transform  TranslationMethod=Cartesian  TranslationLengthUnit=mm  TranslationStandardAxis=+Z  TranslationStandardOffset=0  TranslationCartesianOffset=[-16.089268306127405 -199.74103840837577 40.64935139290418]  TranslationROffset=0  TranslationROffsetUnits=m  TranslationZOffset=0  TranslationZOffsetUnits=m  TranslationThetaOffset=0  TranslationThetaOffsetUnits=deg  RotationMethod=ArbitraryAxis  RotationAngleUnits=rad  RotationStandardAxis=+Z  RotationAngle=2.7352803968007873  RotationArbitraryAxis=[0.20599796797350467 0.69194105138761164 -0.69194105138761164]  FollAlignAxisA=+X  BaseAlignAxisA=+Y  FollAlignAxisB=+Y  BaseAlignAxisB=+Z  BlockFunction=simmechanics.library.frames_transforms.rigid_transform
  Transform6 : sm_lib/Frames and Transforms/Rigid Transform  TranslationMethod=Cartesian  TranslationLengthUnit=mm  TranslationStandardAxis=+Z  TranslationStandardOffset=0  TranslationCartesianOffset=[-16.089268306127405 11.758961591624317 40.64935139290418]  TranslationROffset=0  TranslationROffsetUnits=m  TranslationZOffset=0  TranslationZOffsetUnits=m  TranslationThetaOffset=0  TranslationThetaOffsetUnits=deg  RotationMethod=None  RotationAngleUnits=deg  RotationStandardAxis=+Z  RotationAngle=0  RotationArbitraryAxis=[0 0 1]  FollAlignAxisA=+X  BaseAlignAxisA=+Y  FollAlignAxisB=+Y  BaseAlignAxisB=+Z  BlockFunction=simmechanics.library.frames_transforms.rigid_transform
  uniball_Cuerpo_1_RIGID : Subsystem
  uniball_Cuerpo_2_RIGID : Subsystem
  F : PMIOPort  Port=1  Side=Left
  F1 : PMIOPort  Port=2  Side=Right
  connections:
  ReferenceFrame/RConn1 -- Transform/LConn1 -- Transform1/LConn1 -- Transform2/LConn1 -- Transform3/LConn1 -- Transform4/LConn1 -- Transform5/LConn1 -- Transform6/LConn1
  Transform/RConn1 -- F/RConn1
  Transform1/RConn1 -- F1/RConn1
  Acople_Antebrazo_RUniball_2_RIGID/LConn1 -- Transform2/RConn1
  Antebrazo_1_RIGID/LConn1 -- Transform3/RConn1
  Transform4/RConn1 -- uniball_Cuerpo_2_RIGID/LConn1
  Acople_Antebrazo_RUniball_1_RIGID/LConn1 -- Transform5/RConn1
  Transform6/RConn1 -- uniball_Cuerpo_1_RIGID/LConn1

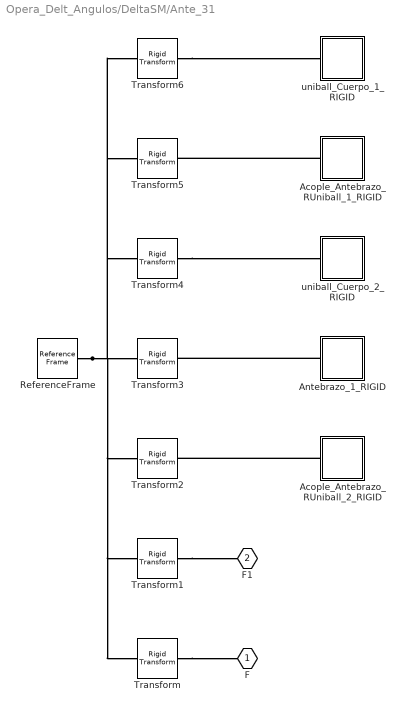
== system Opera_Delt_Angulos/DeltaSM/Ante_31 ==
  Acople_Antebrazo_RUniball_1_RIGID : Subsystem
  Acople_Antebrazo_RUniball_2_RIGID : Subsystem
  Antebrazo_1_RIGID : Subsystem
  ReferenceFrame : sm_lib/Frames and Transforms/Reference Frame  BlockFunction=simmechanics.library.frames_transforms.reference_frame
  Transform : sm_lib/Frames and Transforms/Rigid Transform  TranslationMethod=Cartesian  TranslationLengthUnit=mm  TranslationStandardAxis=+Z  TranslationStandardOffset=0  TranslationCartesianOffset=[-16.089268306127362 11.758961591624349 40.649351392904215]  TranslationROffset=0  TranslationROffsetUnits=m  TranslationZOffset=0  TranslationZOffsetUnits=m  TranslationThetaOffset=0  TranslationThetaOffsetUnits=deg  RotationMethod=ArbitraryAxis  RotationAngleUnits=rad  RotationStandardAxis=+Z  RotationAngle=0  RotationArbitraryAxis=[0 0 0]  FollAlignAxisA=+X  BaseAlignAxisA=+Y  FollAlignAxisB=+Y  BaseAlignAxisB=+Z  BlockFunction=simmechanics.library.frames_transforms.rigid_transform
  Transform1 : sm_lib/Frames and Transforms/Rigid Transform  TranslationMethod=Cartesian  TranslationLengthUnit=mm  TranslationStandardAxis=+Z  TranslationStandardOffset=0  TranslationCartesianOffset=[-16.089268306127391 -263.24103840837569 40.649351392904222]  TranslationROffset=0  TranslationROffsetUnits=m  TranslationZOffset=0  TranslationZOffsetUnits=m  TranslationThetaOffset=0  TranslationThetaOffsetUnits=deg  RotationMethod=ArbitraryAxis  RotationAngleUnits=rad  RotationStandardAxis=+Z  RotationAngle=0  RotationArbitraryAxis=[0 0 0]  FollAlignAxisA=+X  BaseAlignAxisA=+Y  FollAlignAxisB=+Y  BaseAlignAxisB=+Z  BlockFunction=simmechanics.library.frames_transforms.rigid_transform
  Transform2 : sm_lib/Frames and Transforms/Rigid Transform  TranslationMethod=Cartesian  TranslationLengthUnit=mm  TranslationStandardAxis=+Z  TranslationStandardOffset=0  TranslationCartesianOffset=[-16.089268306127376 -51.741038408375701 40.649351392904194]  TranslationROffset=0  TranslationROffsetUnits=m  TranslationZOffset=0  TranslationZOffsetUnits=m  TranslationThetaOffset=0  TranslationThetaOffsetUnits=deg  RotationMethod=ArbitraryAxis  RotationAngleUnits=rad  RotationStandardAxis=+Z  RotationAngle=2.7352803968007873  RotationArbitraryAxis=[-0.20599796797350475 0.69194105138761153 0.69194105138761164]  FollAlignAxisA=+X  BaseAlignAxisA=+Y  FollAlignAxisB=+Y  BaseAlignAxisB=+Z  BlockFunction=simmechanics.library.frames_transforms.rigid_transform
  Transform3 : sm_lib/Frames and Transforms/Rigid Transform  TranslationMethod=Cartesian  TranslationLengthUnit=mm  TranslationStandardAxis=+Z  TranslationStandardOffset=0  TranslationCartesianOffset=[-16.089268306127405 -227.74103840837572 40.649351392904194]  TranslationROffset=0  TranslationROffsetUnits=m  TranslationZOffset=0  TranslationZOffsetUnits=m  TranslationThetaOffset=0  TranslationThetaOffsetUnits=deg  RotationMethod=ArbitraryAxis  RotationAngleUnits=rad  RotationStandardAxis=+Z  RotationAngle=2.7352803968007873  RotationArbitraryAxis=[-0.20599796797350475 0.69194105138761153 0.69194105138761164]  FollAlignAxisA=+X  BaseAlignAxisA=+Y  FollAlignAxisB=+Y  BaseAlignAxisB=+Z  BlockFunction=simmechanics.library.frames_transforms.rigid_transform
  Transform4 : sm_lib/Frames and Transforms/Rigid Transform  TranslationMethod=Cartesian  TranslationLengthUnit=mm  TranslationStandardAxis=+Z  TranslationStandardOffset=0  TranslationCartesianOffset=[-16.089268306127391 -263.24103840837569 40.649351392904222]  TranslationROffset=0  TranslationROffsetUnits=m  TranslationZOffset=0  TranslationZOffsetUnits=m  TranslationThetaOffset=0  TranslationThetaOffsetUnits=deg  RotationMethod=ArbitraryAxis  RotationAngleUnits=rad  RotationStandardAxis=+Z  RotationAngle=3.1415926535897931  RotationArbitraryAxis=[-1.1102230246251565e-16 0 1]  FollAlignAxisA=+X  BaseAlignAxisA=+Y  FollAlignAxisB=+Y  BaseAlignAxisB=+Z  BlockFunction=simmechanics.library.frames_transforms.rigid_transform
  Transform5 : sm_lib/Frames and Transforms/Rigid Transform  TranslationMethod=Cartesian  TranslationLengthUnit=mm  TranslationStandardAxis=+Z  TranslationStandardOffset=0  TranslationCartesianOffset=[-16.089268306127376 -199.74103840837572 40.649351392904208]  TranslationROffset=0  TranslationROffsetUnits=m  TranslationZOffset=0  TranslationZOffsetUnits=m  TranslationThetaOffset=0  TranslationThetaOffsetUnits=deg  RotationMethod=ArbitraryAxis  RotationAngleUnits=rad  RotationStandardAxis=+Z  RotationAngle=2.7352803968007873  RotationArbitraryAxis=[0.20599796797350475 0.69194105138761153 -0.69194105138761164]  FollAlignAxisA=+X  BaseAlignAxisA=+Y  FollAlignAxisB=+Y  BaseAlignAxisB=+Z  BlockFunction=simmechanics.library.frames_transforms.rigid_transform
  Transform6 : sm_lib/Frames and Transforms/Rigid Transform  TranslationMethod=Cartesian  TranslationLengthUnit=mm  TranslationStandardAxis=+Z  TranslationStandardOffset=0  TranslationCartesianOffset=[-16.089268306127405 11.758961591624331 40.649351392904208]  TranslationROffset=0  TranslationROffsetUnits=m  TranslationZOffset=0  TranslationZOffsetUnits=m  TranslationThetaOffset=0  TranslationThetaOffsetUnits=deg  RotationMethod=None  RotationAngleUnits=deg  RotationStandardAxis=+Z  RotationAngle=0  RotationArbitraryAxis=[0 0 1]  FollAlignAxisA=+X  BaseAlignAxisA=+Y  FollAlignAxisB=+Y  BaseAlignAxisB=+Z  BlockFunction=simmechanics.library.frames_transforms.rigid_transform
  uniball_Cuerpo_1_RIGID : Subsystem
  uniball_Cuerpo_2_RIGID : Subsystem
  F : PMIOPort  Port=1  Side=Left
  F1 : PMIOPort  Port=2  Side=Right
  connections:
  ReferenceFrame/RConn1 -- Transform/LConn1 -- Transform1/LConn1 -- Transform2/LConn1 -- Transform3/LConn1 -- Transform4/LConn1 -- Transform5/LConn1 -- Transform6/LConn1
  Transform/RConn1 -- F/RConn1
  Transform1/RConn1 -- F1/RConn1
  Acople_Antebrazo_RUniball_2_RIGID/LConn1 -- Transform2/RConn1
  Antebrazo_1_RIGID/LConn1 -- Transform3/RConn1
  Transform4/RConn1 -- uniball_Cuerpo_2_RIGID/LConn1
  Acople_Antebrazo_RUniball_1_RIGID/LConn1 -- Transform5/RConn1
  Transform6/RConn1 -- uniball_Cuerpo_1_RIGID/LConn1

== matlab function Opera_Delt_Angulos/Posicion  ==
  data: PosX output; PosY output; PosZ output; time input
% function [PosX,PosY,PosZ] = Trayectoria(time)
% 
% 
% TIni=0;
% 
% tf1=2;
% tf2=4;
% tf3=2;
% tf4=2;
% 
% px2i=-40;
% px2f=40;
% 
% pz1i=240;
% pz1f=170;
% 
% pz3i=pz1f;
% pz3f=pz1i;
% 
% pz4i=pz3f;
% pz4f=141.65;
% 
% % %%%%%%%%%%%%%%%%%%%%%%%%%%% funcion Z1
% a10z = pz1i;
% a11z = 0; %velocidad inicial
% a12z = 0; %aceleracion inicial
% a13z = (10*(pz1f-pz1i))/tf1^3;
% a14z = -(15*(pz1f-pz1i))/tf1^4;
% a15z = (6*(pz1f-pz1i))/tf1^5;
% %  z1(t) = a10z + a11z*t + a12z*t^2 + a13z*t^3 + a14z*t^4 + a15z*t^5;
% 
% % %%%%%%%%%%%%%%%%%%%%%%%%%%% funcion Z3
% a30z = pz3i;
% a31z = 0; %velocidad inicial
% a32z = 0; %aceleracion inicial
% a33z = (10*(pz3f-pz3i))/tf3^3;
% a34z = -(15*(pz3f-pz3i))/tf3^4;
% a35z = (6*(pz3f-pz3i))/tf3^5;
% % z3(t) = a30z + a31z*t + a32z*t^2 + a33z*t^3 + a34z*t^4 + a35z*t^5;
% 
% 
% % %%%%%%%%%%%%%%%%%%%%%%%% funcion X2
% a10x = px2i;
% a11x = 0; %velocidad inicial
% a12x = 0; %aceleracion inicial
% a13x = (10*(px2f-px2i))/tf2^3;
% a14x = -(15*(px2f-px2i))/tf2^4;
% a15x = (6*(px2f-px2i))/tf2^5;
% 
% 
% % %%%%%%%%%%%%%%%%%%%%%%%%%%% funcion Z4
% a40z = pz4i;
% a41z = 0; %velocidad inicial
% a42z = 0; %aceleracion inicial
% a43z = (10*(pz4f-pz4i))/tf4^3;
% a44z = -(15*(pz4f-pz4i))/tf4^4;
% a45z = (6*(pz4f-pz4i))/tf3^5;
% % z3(t) = a30z + a31z*t + a32z*t^2 + a33z*t^3 + a34z*t^4 + a35z*t^5;
% 
% % x2(t) = a10x + a11x*t + a12x*t^2 + a13x*t^3 + a14x*t^4 + a15x*t^5;
% % if(time<=TIni)
% %   PosX=0;
% %   PosY=px2i;
% %   PosZ=170;
% if(time<tf1+TIni)
%   tiempo=time-TIni;
%   PosX=0;
%   PosY=px2i;
%   PosZ=a10z + a11z*tiempo + a12z*tiempo^2 + a13z*tiempo^3 + a14z*tiempo^4 + a15z*tiempo^5;
% elseif (time<tf2+tf1+TIni)
%   tiempo=time-tf1-TIni;
%   PosX=0;
%   PosY= a10x + a11x*tiempo + a12x*tiempo^2 + a13x*tiempo^3 + a14x*tiempo^4 + a15x*tiempo^5;
%   PosZ=pz1f;
% 
% elseif (time<tf2+tf1+tf3+TIni)
%   tiempo=time-tf2-tf1-TIni;
%   PosX=0;
%   PosY=px2f;
%   PosZ=a30z + a31z*tiempo + a32z*tiempo^2 + a33z*tiempo^3 + a34z*tiempo^4 + a35z*tiempo^5;
% elseif (time<tf2+tf1+tf3+TIni+tf4)
%   tiempo=time-tf2-tf1-TIni-tf3;
%   PosX=0;
%   PosY=px2f;
%   PosZ=a40z + a41z*tiempo + a42z*tiempo^2 + a43z*tiempo^3 + a44z*tiempo^4 + a45z*tiempo^5;
% else
%   tiempo=tf4;
%   PosX=0;
%   PosY=px2f;
%   PosZ=a40z + a41z*tiempo + a42z*tiempo^2 + a43z*tiempo^3 + a44z*tiempo^4 + a45z*tiempo^5;
% end


% 
function [PosX,PosY,PosZ] = Trayectoria(time)


TIni=0;

tf1=1;
tf2=1;
tf3=1;

% px2i=-20;
% px2f=40;
px2i=-70;
px2f=70;


pz1i=-300;
pz1f=-160;

pz3i=pz1f;
pz3f=-300;


% %%%%%%%%%%%%%%%%%%%%%%%%%%% funcion Z1
a10z = pz1i;
a11z = 0; %velocidad inicial
a12z = 0; %aceleracion inicial
a13z = (10*(pz1f-pz1i))/tf1^3;
a14z = -(15*(pz1f-pz1i))/tf1^4;
a15z = (6*(pz1f-pz1i))/tf1^5;
%  z1(t) = a10z + a11z*t + a12z*t^2 + a13z*t^3 + a14z*t^4 + a15z*t^5;

% %%%%%%%%%%%%%%%%%%%%%%%%%%% funcion Z3
a30z = pz3i;
a31z = 0; %velocidad inicial
a32z = 0; %aceleracion inicial
a33z = (10*(pz3f-pz3i))/tf3^3;
a34z = -(15*(pz3f-pz3i))/tf3^4;
a35z = (6*(pz3f-pz3i))/tf3^5;
% z3(t) = a30z + a31z*t + a32z*t^2 + a33z*t^3 + a34z*t^4 + a35z*t^5;


% %%%%%%%%%%%%%%%%%%%%%%%% funcion X2
a10x = px2i;
a11x = 0; %velocidad inicial
a12x = 0; %aceleracion inicial
a13x = (10*(px2f-px2i))/tf2^3;
a14x = -(15*(px2f-px2i))/tf2^4;
a15x = (6*(px2f-px2i))/tf2^5;
% x2(t) = a10x + a11x*t + a12x*t^2 + a13x*t^3 + a14x*t^4 + a15x*t^5;
% if(time<=TIni)
%   PosX=0;
%   PosY=px2i;
%   PosZ=170;
if(time<tf1+TIni)
  tiempo=time-TIni;
  PosX=0;
  PosY=px2i;
  PosZ=a10z + a11z*tiempo + a12z*tiempo^2 + a13z*tiempo^3 + a14z*tiempo^4 + a15z*tiempo^5;
elseif (time<tf2+tf1+TIni)
  tiempo=time-tf1-TIni;
  PosX=0;
  PosY= a10x + a11x*tiempo + a12x*tiempo^2 + a13x*tiempo^3 + a14x*tiempo^4 + a15x*tiempo^5;
  PosZ=pz1f;

elseif (time<tf2+tf1+tf3+TIni)
  tiempo=time-tf2-tf1-TIni;
  PosX=0;
  PosY=px2f;
  PosZ=a30z + a31z*tiempo + a32z*tiempo^2 + a33z*tiempo^3 + a34z*tiempo^4 + a35z*tiempo^5;
else
  tiempo=tf3;
  PosX=0;
  PosY=px2f;
  PosZ=a30z + a31z*tiempo + a32z*tiempo^2 + a33z*tiempo^3 + a34z*tiempo^4 + a35z*tiempo^5;
end


%
